simulink subsystem "model_2dof_gravity"  (R2020b)
settings: Solver=VariableStepAuto  StartTime=0.0  StopTime=10.0  RelTol=1e-3
values from neighbouring files (symbols this model uses):
  cr = 2*sqrt(kr*mr)    [main.m]    (also in state_function.m)
  g = 9.81    [main.m]    (also in state_function.m)
  Jy = (mf*Lf^2)/3    (= 312915.96)    [main.m]    (also in state_function.m)
  kf = 1e6    (= 1000000)    [main.m]    (also in state_function.m)
  kr = 1e6    (= 1000000)    [main.m]    (also in state_function.m)
  ktf = 2.1e6    (= 2100000)    [main.m]    (also in state_function.m)
  ktr = 2.1e6    (= 2100000)    [main.m]    (also in state_function.m)
  Lf = L*0.90    (= 11.34)    [main.m]    (also in state_function.m)
  Lr = L-Lf    (= 1.26)    [main.m]    (also in state_function.m)
  M = 73000    [main.m]    (also in state_function.m)
  mtf = 120*2    (= 240)    [main.m]    (also in state_function.m)
  mtr = 120*8    (= 960)    [main.m]    (also in state_function.m)
  theta0 = (pi/180)*2    (= 0.0349065850399)    [main.m]
  z0 = 50    [main.m]
  zwf0 = z0+Lf*sin(theta0)-((mtf*g/kf)+L0)    [main.m]
  zwr0 = z0-Lr*sin(theta0)-((mtr*g/kr)+L0)    [main.m]
settings Model: Creator=alema  LastModifiedBy=alema

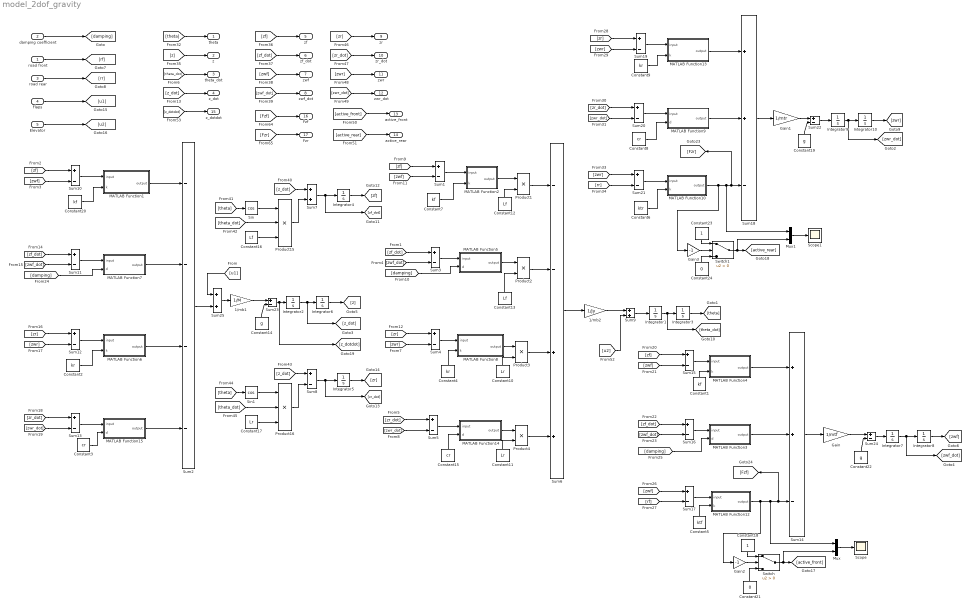
== system model_2dof_gravity ==
  road front : Inport
  damping coefficient : Inport  Port=2
  road rear : Inport  Port=3
  Flaps : Inport  Port=4
  Elevator : Inport  Port=5
  1/mb1 : Gain  Gain=1/M
  1/mb2 : Gain  Gain=1/Jy
  Constant1 : Constant  Value=kf
  Constant10 : Constant  Value=Lr
  Constant11 : Constant  Value=Lr
  Constant12 : Constant  Value=Lf
  Constant13 : Constant  Value=Lf
  Constant14 : Constant  Value=g
  Constant15 : Constant  Value=cr
  Constant16 : Constant  Value=Lf
  Constant17 : Constant  Value=Lr
  Constant18 : Constant
  Constant19 : Constant  Value=g
  Constant2 : Constant  Value=kr
  Constant20 : Constant  Value=kf
  Constant21 : Constant  Value=0
  Constant22 : Constant  Value=g
  Constant23 : Constant
  Constant24 : Constant  Value=0
  Constant3 : Constant  Value=cr
  Constant4 : Constant  Value=kr
  Constant5 : Constant  Value=ktf
  Constant6 : Constant  Value=ktr
  Constant7 : Constant  Value=kf
  Constant8 : Constant  Value=cr
  Constant9 : Constant  Value=kr
  Gain : Gain  Gain=1/mtf
  Gain1 : Gain  Gain=1/mtr
  Gain2 : Gain  Gain=-1
  Gain3 : Gain  Gain=-1
  Integrator{1..2,7,9} (4 alike) : Integrator
  Integrator10 : Integrator  InitialCondition=zwr0
  Integrator3 : Integrator  InitialCondition=theta0
  Integrator4 : Integrator  InitialCondition=z0+Lf*sin(theta0)
  Integrator5 : Integrator  InitialCondition=z0-Lr*sin(theta0)
  Integrator6 : Integrator  InitialCondition=z0
  Integrator8 : Integrator  InitialCondition=zwf0
  MATLAB Function1 : MATLAB Function  TreatAsAtomicUnit=on
  MATLAB Function10 : MATLAB Function  TreatAsAtomicUnit=on
  MATLAB Function12 : MATLAB Function  TreatAsAtomicUnit=on
  MATLAB Function13 : MATLAB Function  TreatAsAtomicUnit=on
  MATLAB Function14 : MATLAB Function  TreatAsAtomicUnit=on
  MATLAB Function15 : MATLAB Function  TreatAsAtomicUnit=on
  MATLAB Function2 : MATLAB Function  TreatAsAtomicUnit=on
  MATLAB Function3 : MATLAB Function  TreatAsAtomicUnit=on
  MATLAB Function4 : MATLAB Function  TreatAsAtomicUnit=on
  MATLAB Function5 : MATLAB Function  TreatAsAtomicUnit=on
  MATLAB Function6 : MATLAB Function  TreatAsAtomicUnit=on
  MATLAB Function7 : MATLAB Function  TreatAsAtomicUnit=on
  MATLAB Function8 : MATLAB Function  TreatAsAtomicUnit=on
  MATLAB Function9 : MATLAB Function  TreatAsAtomicUnit=on
  Mux : Mux  Inputs=2
  Mux1 : Mux  Inputs=2
  Product{1..4} (4 alike) : Product
  Product15 : Product  Inputs=3
  Product16 : Product  Inputs=3
  Scope : Scope
  Scope1 : Scope
  Sin : Trigonometry  Operator=cos
  Sin1 : Trigonometry  Operator=cos
  Sum{1,3..5,8,10..13,15..17,19..24} (18 alike) : Sum  Inputs=+-
  Sum14 : Sum  Inputs=++-
  Sum18 : Sum  Inputs=++-
  Sum2 : Sum  Inputs=----
  Sum25 : Sum
  Sum6 : Sum  Inputs=--++
  Sum7 : Sum
  Sum9 : Sum
  Switch : Switch  Criteria=u2 > Threshold
  Switch1 : Switch  Criteria=u2 > Threshold
  theta : Outport
  z : Outport  Port=2
  theta_dot : Outport  Port=3
  z_dot : Outport  Port=4
  zf : Outport  Port=5
  zf_dot : Outport  Port=6
  zwf : Outport  Port=7
  zwf_dot : Outport  Port=8
  zr : Outport  Port=9
  zr_dot : Outport  Port=10
  zwr : Outport  Port=11
  zwr_dot : Outport  Port=12
  active_front : Outport  Port=13
  active_rear : Outport  Port=14
  z_dotdot : Outport  Port=15
  Fzf : Outport  Port=16
  Fzr : Outport  Port=17
  wires:
  Integrator2/1 -> Integrator6/1, [z_dot]
  Integrator6/1 -> [z]
  Sum10/1 -> MATLAB Function1/1(input)
  [zwf] -> Sum10/2
  [zf] -> Sum10/1
  MATLAB Function1/1(output) -> Sum2/1
  [zwf_dot] -> Sum11/2
  [zf_dot] -> Sum11/1
  Sum11/1 -> MATLAB Function7/1(input)
  MATLAB Function7/1(output) -> Sum2/2
  [zwr] -> Sum12/2
  [zr] -> Sum12/1
  Sum12/1 -> MATLAB Function6/1(input)
  MATLAB Function6/1(output) -> Sum2/3
  [zr_dot] -> Sum13/1
  [zwr_dot] -> Sum13/2
  Sum13/1 -> MATLAB Function15/1(input)
  MATLAB Function15/1(output) -> Sum2/4
  Integrator7/1 -> Integrator8/1, [zwf_dot]
  Integrator8/1 -> [zwf]
  Sum14/1 -> Gain/1
  [zwf] -> Sum15/2
  [zf] -> Sum15/1
  [zwf_dot] -> Sum16/2
  [zf_dot] -> Sum16/1
  Sum16/1 -> MATLAB Function3/1(input)
  damping coefficient/1 -> [damping]
  [damping] -> MATLAB Function7/2(d)
  MATLAB Function12/1(output) -> Gain2/1, Mux/1, Sum14/3, [Fzf]
  [rf] -> Sum17/2
  [zwf] -> Sum17/1
  Sum17/1 -> MATLAB Function12/1(input)
  road front/1 -> [rf]
  road rear/1 -> [rr]
  MATLAB Function13/1(output) -> Sum18/1
  [zwr] -> Sum21/1
  [rr] -> Sum21/2
  Sum20/1 -> MATLAB Function9/1(input)
  [zr_dot] -> Sum20/1
  [zwr_dot] -> Sum20/2
  Sum21/1 -> MATLAB Function10/1(input)
  [zwr] -> Sum19/2
  [zr] -> Sum19/1
  Sum19/1 -> MATLAB Function13/1(input)
  Integrator10/1 -> [zwr]
  Sum18/1 -> Gain1/1
  MATLAB Function9/1(output) -> Sum18/2
  Integrator9/1 -> Integrator10/1, [zwr_dot]
  Product1/1 -> Sum6/1
  [zf] -> Sum1/1
  [zwf] -> Sum1/2
  [zf_dot] -> Sum3/1
  [zwf_dot] -> Sum3/2
  Sum6/1 -> 1/mb2/1
  Product2/1 -> Sum6/2
  Sum1/1 -> MATLAB Function2/1(input)
  Product4/1 -> Sum6/4
  [zwr_dot] -> Sum5/2
  [zr] -> Sum4/1
  [zwr] -> Sum4/2
  Product3/1 -> Sum6/3
  [zr_dot] -> Sum5/1
  Sum5/1 -> MATLAB Function14/1(input)
  [theta] -> theta/1
  [z] -> z/1
  [zf] -> zf/1
  [zf_dot] -> zf_dot/1
  [zwf] -> zwf/1
  [zwf_dot] -> zwf_dot/1
  [theta_dot] -> theta_dot/1
  [z_dot] -> z_dot/1
  Integrator4/1 -> [zf]
  [z_dot] -> Sum7/1
  Product15/1 -> Sum7/2
  Sin/1 -> Product15/1
  [theta] -> Sin/1
  Sum7/1 -> Integrator4/1, [zf_dot]
  [theta_dot] -> Product15/2
  Constant16/1 -> Product15/3
  Sin1/1 -> Product16/1
  Product16/1 -> Sum8/2
  [theta_dot] -> Product16/2
  [theta] -> Sin1/1
  [z_dot] -> Sum8/1
  Sum8/1 -> Integrator5/1, [zr_dot]
  Constant17/1 -> Product16/3
  Integrator5/1 -> [zr]
  Gain1/1 -> Sum22/1
  Constant19/1 -> Sum22/2
  Sum22/1 -> Integrator9/1
  [zwr] -> zwr/1
  [zwr_dot] -> zwr_dot/1
  [zr_dot] -> zr_dot/1
  [zr] -> zr/1
  Constant9/1 -> MATLAB Function13/2(k)
  Constant20/1 -> MATLAB Function1/2(k)
  Constant2/1 -> MATLAB Function6/2(k)
  Constant7/1 -> MATLAB Function2/2(k)
  MATLAB Function2/1(output) -> Product1/1
  Constant12/1 -> Product1/2
  Sum4/1 -> MATLAB Function8/1(input)
  Constant4/1 -> MATLAB Function8/2(k)
  MATLAB Function8/1(output) -> Product3/1
  Constant10/1 -> Product3/2
  Sum15/1 -> MATLAB Function4/1(input)
  MATLAB Function4/1(output) -> Sum14/1
  Constant1/1 -> MATLAB Function4/2(k)
  Constant5/1 -> MATLAB Function12/2(k)
  Constant6/1 -> MATLAB Function10/2(k)
  Constant3/1 -> MATLAB Function15/2(d)
  Constant8/1 -> MATLAB Function9/2(d)
  Constant15/1 -> MATLAB Function14/2(d)
  MATLAB Function14/1(output) -> Product4/1
  Constant11/1 -> Product4/2
  Sum3/1 -> MATLAB Function5/1(input)
  MATLAB Function5/1(output) -> Product2/1
  [damping] -> MATLAB Function5/2(d)
  Constant13/1 -> Product2/2
  MATLAB Function3/1(output) -> Sum14/2
  [damping] -> MATLAB Function3/2(d)
  Flaps/1 -> [u1]
  Elevator/1 -> [u2]
  Constant22/1 -> Sum24/2
  Gain/1 -> Sum24/1
  Sum24/1 -> Integrator7/1
  [u2] -> Sum9/2
  1/mb2/1 -> Sum9/1
  Integrator1/1 -> Integrator3/1, [theta_dot]
  Integrator3/1 -> [theta]
  Sum9/1 -> Integrator1/1
  [active_front] -> active_front/1
  Constant18/1 -> Switch/1
  Switch/1 -> [active_front], Mux/2
  Mux/1 -> Scope/1
  Constant21/1 -> Switch/3
  Gain2/1 -> Switch/2
  Constant14/1 -> Sum23/2
  Sum23/1 -> Integrator2/1, [z_dotdot]
  1/mb1/1 -> Sum23/1
  Sum2/1 -> Sum25/2
  Sum25/1 -> 1/mb1/1
  [u1] -> Sum25/1
  Constant24/1 -> Switch1/3
  Mux1/1 -> Scope1/1
  Constant23/1 -> Switch1/1
  Gain3/1 -> Switch1/2
  MATLAB Function10/1(output) -> Mux1/1, Sum18/3, [Fzr], Gain3/1
  Switch1/1 -> [active_rear], Mux1/2
  [active_rear] -> active_rear/1
  [z_dotdot] -> z_dotdot/1
  [Fzf] -> Fzf/1
  [Fzr] -> Fzr/1

== matlab function model_2dof_gravity/MATLAB Function14 ==
  data: input input; output output; d input
function output = function_fda(input,d)
    output=fda(input,d);
end

== matlab function model_2dof_gravity/MATLAB Function15 ==
  data: input input; output output; d input
function output = function_fda(input,d)
    output=fda(input,d);
end

== matlab function model_2dof_gravity/MATLAB Function3 ==
  data: input input; output output; d input
function output = function_fda(input,d)
    output=fda(input,d);
end

== matlab function model_2dof_gravity/MATLAB Function4 ==
  data: input input; output output; k input
function output = function_fel(input,k)
    output=fel(input,k);
end

== matlab function model_2dof_gravity/MATLAB Function5 ==
  data: input input; output output; d input
function output = function_fda(input,d)
    output=fda(input,d);
end

== matlab function model_2dof_gravity/MATLAB Function1 ==
  data: input input; output output; k input
function output = function_fel(input,k)
    output=fel(input,k);
end

== matlab function model_2dof_gravity/MATLAB Function6 ==
  data: input input; output output; k input
function output = function_fel(input,k)
    output=fel(input,k);
end

== matlab function model_2dof_gravity/MATLAB Function7 ==
  data: input input; output output; d input
function output = function_fda(input,d)
    output=fda(input,d);
end

== matlab function model_2dof_gravity/MATLAB Function8 ==
  data: input input; output output; k input
function output = function_fel(input,k)
    output=fel(input,k);
end

== matlab function model_2dof_gravity/MATLAB Function9 ==
  data: input input; output output; d input
function output = function_fda(input,d)
    output=fda(input,d);
end

== matlab function model_2dof_gravity/MATLAB Function10 ==
  data: input input; output output; k input
function output = function_felt(input,k)
    output=felt(input,k);
end

== matlab function model_2dof_gravity/MATLAB Function12 ==
  data: input input; output output; k input
function output = function_felt(input,k)
    output=felt(input,k);
end

== matlab function model_2dof_gravity/MATLAB Function2 ==
  data: input input; output output; k input
function output = function_fel(input,k)
    output=fel(input,k);
end

== matlab function model_2dof_gravity/MATLAB Function13 ==
  data: input input; output output; k input
function output = function_fel(input,k)
    output=fel(input,k);
end
